simulink library "SEMACE2_OUT"  (R2021b)
settings: Solver=VariableStepAuto  StartTime=0.0  StopTime=10.0  RelTol=1e-3
settings Model: Creator=ACH  LastModifiedBy=ACH

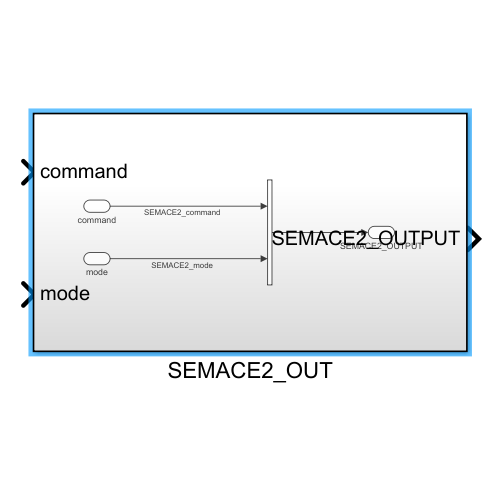
[thumbnail: Simulink's stored preview of the top-level diagram]
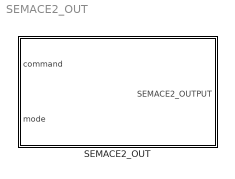
== system SEMACE2_OUT ==
  SEMACE2_OUT : Subsystem

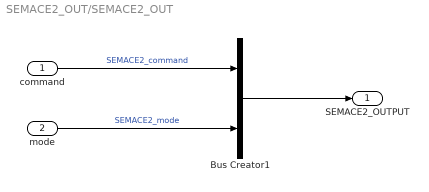
== system SEMACE2_OUT/SEMACE2_OUT ==
  command : Inport
  mode : Inport  Port=2
  Bus Creator1 : BusCreator  Inputs=2  OutDataTypeStr=Bus: SEMACE2_OUTPUT
  SEMACE2_OUTPUT : Outport  OutDataTypeStr=Bus: SEMACE2_OUTPUT
  wires:
  command/1 -> Bus Creator1/1  "SEMACE2_command"
  mode/1 -> Bus Creator1/2  "SEMACE2_mode"
  Bus Creator1/1 -> SEMACE2_OUTPUT/1
